simulink subsystem "ChiefGNC"  (R2023a)
settings: Solver=VariableStepAuto  StartTime=0.0  StopTime=10.0  RelTol=1e-3
undefined symbols (not defined in the file or in its folder): DiscIntNeverNeededParam, nav, satControlData_Rot, satControlData_Trans
settings Model: Creator=Andy  LastModifiedBy=Andy

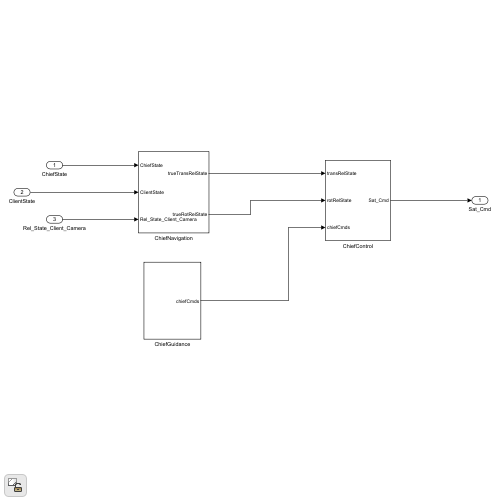
[thumbnail: Simulink's stored preview of the top-level diagram]
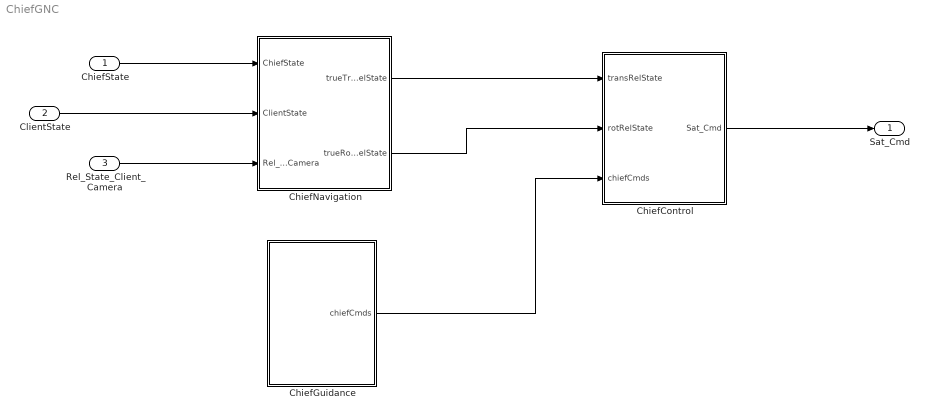
== system ChiefGNC ==
  ChiefState : Inport
  ClientState : Inport  Port=2
  Rel_State_Client_Camera : Inport  Port=3
  ChiefControl : Subsystem
  ChiefGuidance : Subsystem
  ChiefNavigation : Subsystem
  Sat_Cmd : Outport
  wires:
  ChiefGuidance/1(chiefCmds) -> ChiefControl/3(chiefCmds)
  ChiefNavigation/1(trueTransRelState) -> ChiefControl/1(transRelState)
  ChiefState/1 -> ChiefNavigation/1(ChiefState)
  ChiefNavigation/2(trueRotRelState) -> ChiefControl/2(rotRelState)
  ChiefControl/1(Sat_Cmd) -> Sat_Cmd/1
  ClientState/1 -> ChiefNavigation/2(ClientState)
  Rel_State_Client_Camera/1 -> ChiefNavigation/3(Rel_State_Client_Camera)

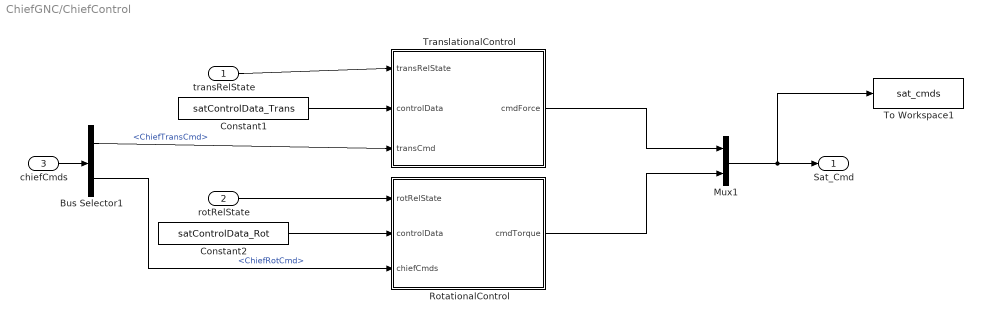
== system ChiefGNC/ChiefControl ==
  transRelState : Inport
  rotRelState : Inport  Port=2
  chiefCmds : Inport  Port=3
  Bus Selector1 : BusSelector  OutputSignals=ChiefTransCmd,ChiefRotCmd
  Constant1 : Constant  Value=satControlData_Trans  OutDataTypeStr=Bus: satControlDataBus_Trans
  Constant2 : Constant  Value=satControlData_Rot  OutDataTypeStr=Bus: satControlDataBus_Rot
  Mux1 : Mux  Inputs=2
  RotationalControl : Subsystem
  To Workspace1 : ToWorkspace  VariableName=sat_cmds  SaveFormat=Timeseries  SampleTime=-1
  TranslationalControl : Subsystem
  Sat_Cmd : Outport
  wires:
  Bus Selector1/2 -> RotationalControl/3(chiefCmds)  "<ChiefRotCmd>"
  Bus Selector1/1 -> TranslationalControl/3(transCmd)  "<ChiefTransCmd>"
  chiefCmds/1 -> Bus Selector1/1
  Mux1/1 -> Sat_Cmd/1, To Workspace1/1
  TranslationalControl/1(cmdForce) -> Mux1/1
  Constant1/1 -> TranslationalControl/2(controlData)
  Constant2/1 -> RotationalControl/2(controlData)
  transRelState/1 -> TranslationalControl/1(transRelState)
  RotationalControl/1(cmdTorque) -> Mux1/2
  rotRelState/1 -> RotationalControl/1(rotRelState)

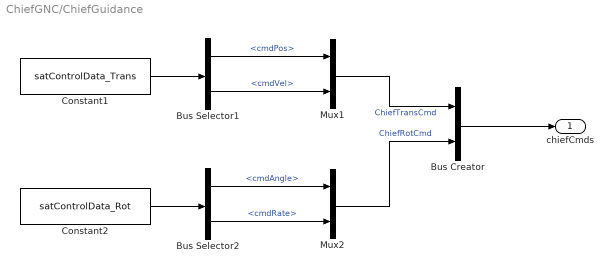
== system ChiefGNC/ChiefGuidance ==
  Bus Creator : BusCreator  Inputs=2
  Bus Selector1 : BusSelector  OutputSignals=cmdPos,cmdVel
  Bus Selector2 : BusSelector  OutputSignals=cmdAngle,cmdRate
  Constant1 : Constant  Value=satControlData_Trans  OutDataTypeStr=Bus: satControlDataBus_Trans
  Constant2 : Constant  Value=satControlData_Rot  OutDataTypeStr=Bus: satControlDataBus_Rot
  Mux1 : Mux  Inputs=2
  Mux2 : Mux  Inputs=2
  chiefCmds : Outport
  wires:
  Bus Creator/1 -> chiefCmds/1
  Mux2/1 -> Bus Creator/2  "ChiefRotCmd"
  Bus Selector2/2 -> Mux2/2  "<cmdRate>"
  Bus Selector1/1 -> Mux1/1  "<cmdPos>"
  Bus Selector1/2 -> Mux1/2  "<cmdVel>"
  Bus Selector2/1 -> Mux2/1  "<cmdAngle>"
  Constant1/1 -> Bus Selector1/1
  Mux1/1 -> Bus Creator/1  "ChiefTransCmd"
  Constant2/1 -> Bus Selector2/1

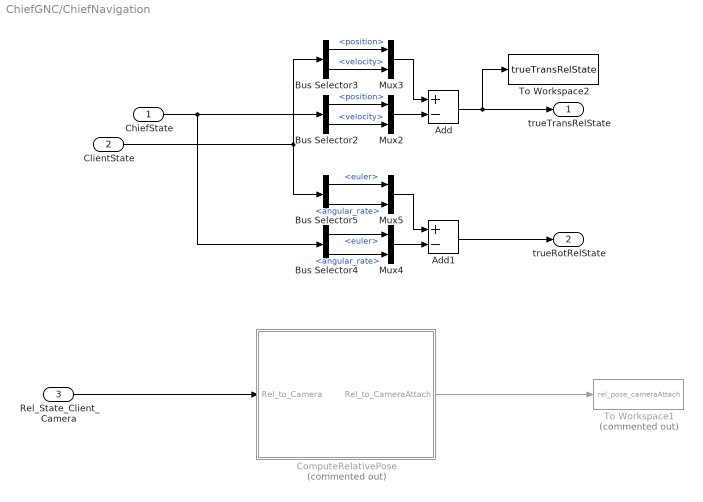
== system ChiefGNC/ChiefNavigation ==
  ChiefState : Inport
  ClientState : Inport  Port=2
  Rel_State_Client_Camera : Inport  Port=3
  Add : Sum  Inputs=+-
  Add1 : Sum  Inputs=+-
  Bus Selector2 : BusSelector  OutputSignals=translation.position,translation.velocity
  Bus Selector3 : BusSelector  OutputSignals=translation.position,translation.velocity
  Bus Selector4 : BusSelector  OutputSignals=rotation.euler,rotation.angular_rate
  Bus Selector5 : BusSelector  OutputSignals=rotation.euler,rotation.angular_rate
  ComputeRelativePose : Subsystem  Commented=on
  Mux{2..5} (4 alike) : Mux  Inputs=2
  To Workspace1 : ToWorkspace  Commented=on  VariableName=rel_pose_cameraAttach  SaveFormat=Timeseries  SampleTime=-1
  To Workspace2 : ToWorkspace  VariableName=trueTransRelState  SaveFormat=Timeseries  SampleTime=-1
  trueTransRelState : Outport
  trueRotRelState : Outport  Port=2
  wires:
  Rel_State_Client_Camera/1 -> ComputeRelativePose/1(Rel_to_Camera)
  ComputeRelativePose/1("Rel_to_CameraAttach ") -> To Workspace1/1
  Bus Selector5/1 -> Mux5/1  "<euler>"
  Bus Selector2/2 -> Mux2/2  "<velocity>"
  Add/1 -> To Workspace2/1, trueTransRelState/1
  Bus Selector2/1 -> Mux2/1  "<position>"
  Mux2/1 -> Add/2
  Bus Selector4/2 -> Mux4/2  "<angular_rate>"
  Mux3/1 -> Add/1
  Bus Selector3/1 -> Mux3/1  "<position>"
  Add1/1 -> trueRotRelState/1
  Bus Selector4/1 -> Mux4/1  "<euler>"
  Bus Selector5/2 -> Mux5/2  "<angular_rate>"
  Bus Selector3/2 -> Mux3/2  "<velocity>"
  Mux4/1 -> Add1/2
  ChiefState/1 -> Bus Selector4/1, Bus Selector2/1
  ClientState/1 -> Bus Selector5/1, Bus Selector3/1
  Mux5/1 -> Add1/1

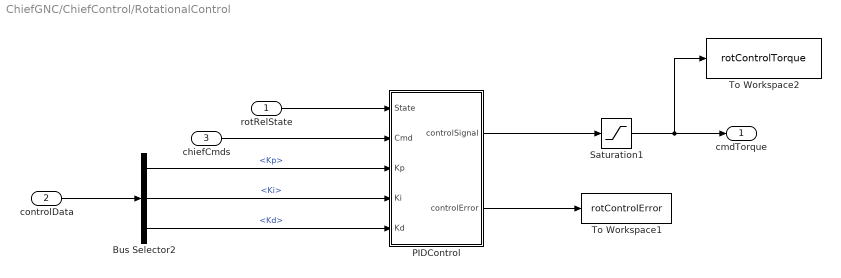
== system ChiefGNC/ChiefControl/RotationalControl ==
  rotRelState : Inport
  controlData : Inport  Port=2
  chiefCmds : Inport  Port=3
  Bus Selector2 : BusSelector  OutputSignals=Kp,Ki,Kd
  PIDControl : Subsystem
  Saturation1 : Saturate  UpperLimit=satControlData_Rot.torqueLimit  LowerLimit=-satControlData_Rot.torqueLimit
  To Workspace1 : ToWorkspace  VariableName=rotControlError  SaveFormat=Timeseries  SampleTime=-1
  To Workspace2 : ToWorkspace  VariableName=rotControlTorque  SaveFormat=Timeseries  SampleTime=-1
  cmdTorque : Outport
  wires:
  chiefCmds/1 -> PIDControl/2(Cmd)
  PIDControl/1(controlSignal) -> Saturation1/1
  Bus Selector2/3 -> PIDControl/5(Kd)  "<Kd>"
  Bus Selector2/2 -> PIDControl/4(Ki)  "<Ki>"
  Bus Selector2/1 -> PIDControl/3(Kp)  "<Kp>"
  controlData/1 -> Bus Selector2/1
  PIDControl/2(controlError) -> To Workspace1/1
  Saturation1/1 -> cmdTorque/1, To Workspace2/1
  rotRelState/1 -> PIDControl/1(State)

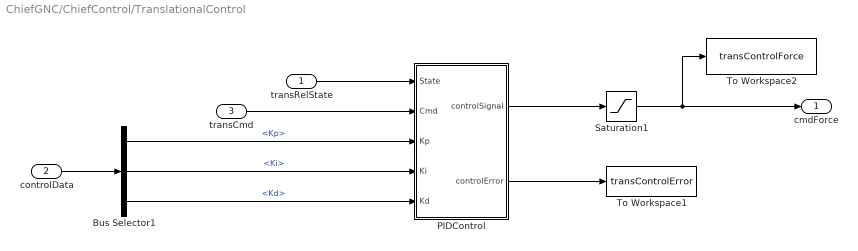
== system ChiefGNC/ChiefControl/TranslationalControl ==
  transRelState : Inport
  controlData : Inport  Port=2
  transCmd : Inport  Port=3
  Bus Selector1 : BusSelector  OutputSignals=Kp,Ki,Kd
  PIDControl : Subsystem
  Saturation1 : Saturate  UpperLimit=satControlData_Trans.forceLimit  LowerLimit=-satControlData_Trans.forceLimit  LinearizeAsGain=off
  To Workspace1 : ToWorkspace  VariableName=transControlError  SaveFormat=Timeseries  SampleTime=-1
  To Workspace2 : ToWorkspace  VariableName=transControlForce  SaveFormat=Timeseries  SampleTime=-1
  cmdForce : Outport
  wires:
  transCmd/1 -> PIDControl/2(Cmd)
  Bus Selector1/3 -> PIDControl/5(Kd)  "<Kd>"
  Bus Selector1/2 -> PIDControl/4(Ki)  "<Ki>"
  Bus Selector1/1 -> PIDControl/3(Kp)  "<Kp>"
  controlData/1 -> Bus Selector1/1
  PIDControl/2(controlError) -> To Workspace1/1
  Saturation1/1 -> To Workspace2/1, cmdForce/1
  PIDControl/1(controlSignal) -> Saturation1/1
  transRelState/1 -> PIDControl/1(State)

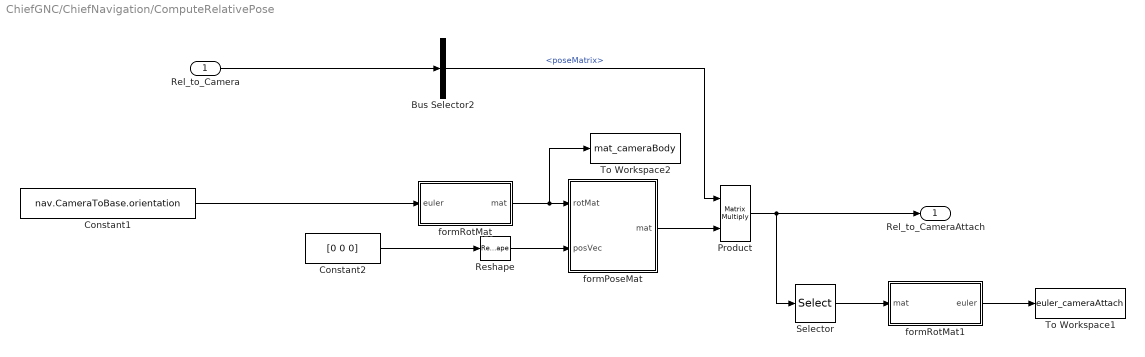
== system ChiefGNC/ChiefNavigation/ComputeRelativePose ==
  Rel_to_Camera : Inport
  Bus Selector2 : BusSelector  OutputSignals=poseMatrix
  Constant1 : Constant  Value=nav.CameraToBase.orientation
  Constant2 : Constant  Value=[0 0 0]
  Product : Product  Multiplication=Matrix(*)
  Reshape : Reshape  OutputDimensionality=Column vector (2-D)
  Selector : Selector  NumberOfDimensions=2  InputPortWidth=3  IndexOptions=Index vector (dialog),Index vector (dialog)  Indices=[1:3],[1:3]  OutputSizes=1,1
  To Workspace1 : ToWorkspace  VariableName=euler_cameraAttach  SaveFormat=Timeseries  SampleTime=-1
  To Workspace2 : ToWorkspace  VariableName=mat_cameraBody  SaveFormat=Timeseries  SampleTime=-1
  formPoseMat : MATLAB Function  TreatAsAtomicUnit=on
  formRotMat : MATLAB Function  TreatAsAtomicUnit=on
  formRotMat1 : MATLAB Function  TreatAsAtomicUnit=on
  "Rel_to_CameraAttach " : Outport
  wires:
  Bus Selector2/1 -> Product/1  "<poseMatrix>"
  formPoseMat/1(mat) -> Product/2
  Constant1/1 -> formRotMat/1(euler)
  Reshape/1 -> formPoseMat/2(posVec)
  Constant2/1 -> Reshape/1
  formRotMat1/1(euler) -> To Workspace1/1
  Selector/1 -> formRotMat1/1(mat)
  Product/1 -> "Rel_to_CameraAttach "/1, Selector/1
  Rel_to_Camera/1 -> Bus Selector2/1
  formRotMat/1(mat) -> formPoseMat/1(rotMat), To Workspace2/1

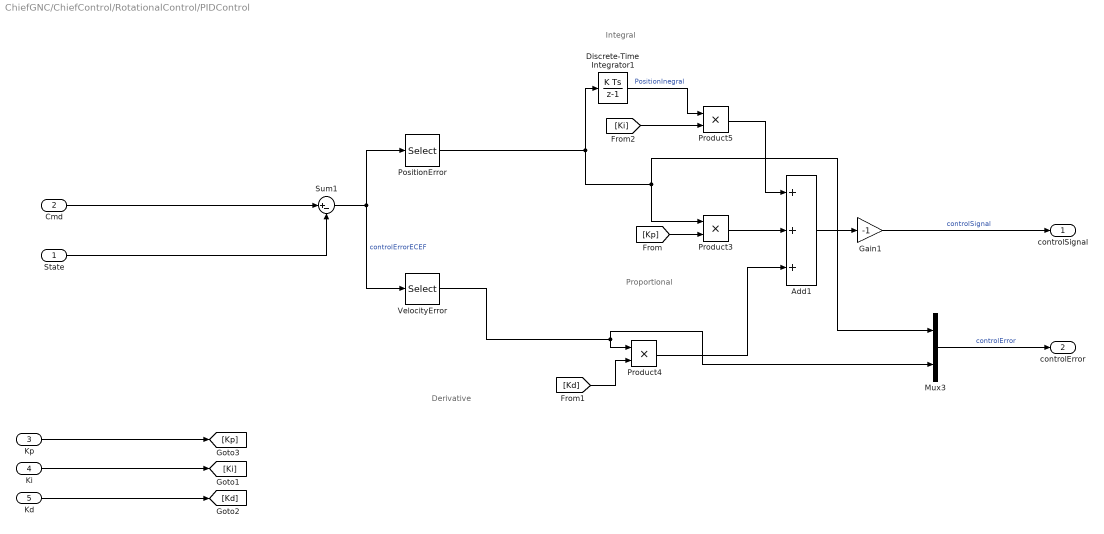
== system ChiefGNC/ChiefControl/RotationalControl/PIDControl ==
  note: Integral
  note: Proportional
  note: Derivative
  State : Inport
  Cmd : Inport  Port=2
  Kp : Inport  Port=3
  Ki : Inport  Port=4
  Kd : Inport  Port=5
  Add1 : Sum  Inputs=+++
  Discrete-Time Integrator1 : DiscreteIntegrator  SampleTime=-1  ICPrevOutput=DiscIntNeverNeededParam  ICPrevScaledInput=DiscIntNeverNeededParam
  Gain1 : Gain  Gain=-1
  Mux3 : Mux  Inputs=2
  PositionError : Selector  IndexOptions=Index vector (dialog)  Indices=[1:3]  OutputSizes=1
  Product3 : Product
  Product4 : Product
  Product5 : Product
  Sum1 : Sum  Inputs=|+-
  VelocityError : Selector  IndexOptions=Index vector (dialog)  Indices=[4:6]  OutputSizes=1
  controlSignal : Outport
  controlError : Outport  Port=2
  wires:
  Ki/1 -> [Ki]
  Kd/1 -> [Kd]
  Kp/1 -> [Kp]
  Cmd/1 -> Sum1/1
  Product4/1 -> Add1/3
  Add1/1 -> Gain1/1
  [Kd] -> Product4/2
  [Kp] -> Product3/2
  [Ki] -> Product5/2
  Mux3/1 -> controlError/1  "controlError"
  VelocityError/1 -> Mux3/2, Product4/1
  Gain1/1 -> controlSignal/1  "controlSignal"
  State/1 -> Sum1/2
  Product5/1 -> Add1/1
  Discrete-Time Integrator1/1 -> Product5/1  "PositionInegral"
  Sum1/1 -> PositionError/1, VelocityError/1  "controlErrorECEF"
  Product3/1 -> Add1/2
  PositionError/1 -> Discrete-Time Integrator1/1, Mux3/1, Product3/1

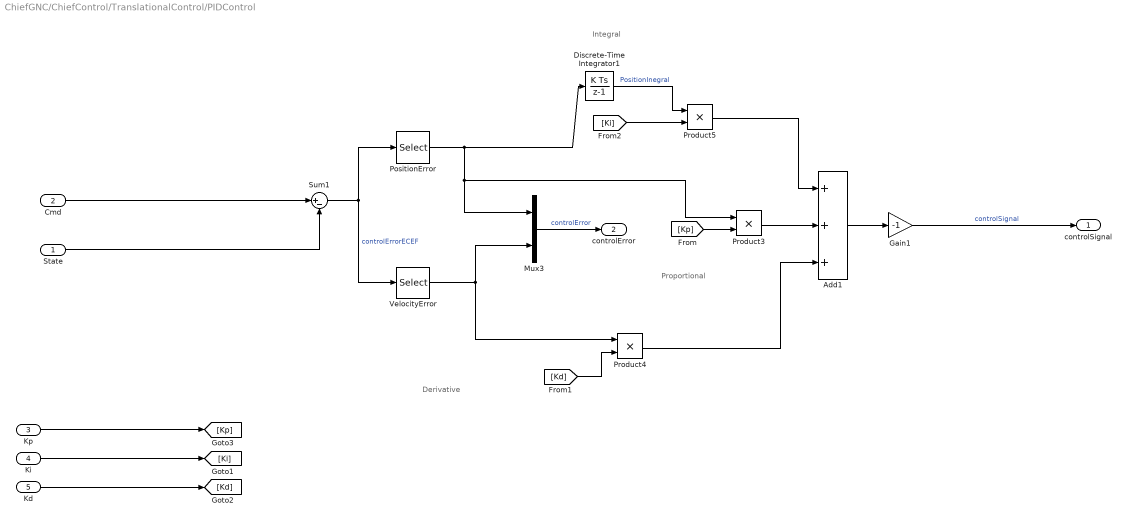
== system ChiefGNC/ChiefControl/TranslationalControl/PIDControl ==
  note: Integral
  note: Proportional
  note: Derivative
  State : Inport
  Cmd : Inport  Port=2
  Kp : Inport  Port=3
  Ki : Inport  Port=4
  Kd : Inport  Port=5
  Add1 : Sum  Inputs=+++
  Discrete-Time Integrator1 : DiscreteIntegrator  SampleTime=-1  ICPrevOutput=DiscIntNeverNeededParam  ICPrevScaledInput=DiscIntNeverNeededParam
  Gain1 : Gain  Gain=-1
  Mux3 : Mux  Inputs=2
  PositionError : Selector  IndexOptions=Index vector (dialog)  Indices=[1:3]  OutputSizes=1
  Product3 : Product
  Product4 : Product
  Product5 : Product
  Sum1 : Sum  Inputs=|+-
  VelocityError : Selector  IndexOptions=Index vector (dialog)  Indices=[4:6]  OutputSizes=1
  controlSignal : Outport
  controlError : Outport  Port=2
  wires:
  Ki/1 -> [Ki]
  Kd/1 -> [Kd]
  Kp/1 -> [Kp]
  Cmd/1 -> Sum1/1
  Product4/1 -> Add1/3
  Add1/1 -> Gain1/1
  [Kd] -> Product4/2
  [Kp] -> Product3/2
  [Ki] -> Product5/2
  Mux3/1 -> controlError/1  "controlError"
  VelocityError/1 -> Mux3/2, Product4/1
  Gain1/1 -> controlSignal/1  "controlSignal"
  State/1 -> Sum1/2
  Product5/1 -> Add1/1
  Discrete-Time Integrator1/1 -> Product5/1  "PositionInegral"
  Sum1/1 -> PositionError/1, VelocityError/1  "controlErrorECEF"
  Product3/1 -> Add1/2
  PositionError/1 -> Mux3/1, Product3/1, Discrete-Time Integrator1/1

== matlab function ChiefGNC/ChiefNavigation/ComputeRelativePose/formPoseMat ==
  data: rotMat input; mat output; posVec input
function mat  = callFormPoseMat(rotMat,posVec)


[mat] = formPoseMat(rotMat,posVec);

== matlab function ChiefGNC/ChiefNavigation/ComputeRelativePose/formRotMat ==
  data: euler input; mat output
function mat  = callEulerToDCM(euler)

[mat] = robotEulerToDCM_321(euler);

== matlab function ChiefGNC/ChiefNavigation/ComputeRelativePose/formRotMat1 ==
  data: mat input; euler output
function euler  = callDCMToEuler(mat)

[euler] = robotDCMToEuler_321(mat);
